simulink model "lqr_control"  (Simulink 8.0)
settings: Solver=FixedStepDiscrete  StartTime=0.0  StopTime=10.0  FixedStep=SampleTime  RelTol=1e-3
undefined symbols (not defined in the file or in its folder): DiscIntNeverNeededParam, K_pitch, K_roll, SampleTime
libraries: simulink x1
settings Model: Creator=austinmurch  LastModifiedBy=brtaylor
settings DataIOCC: SignalLoggingSaveFormat=ModelDataLogs
settings OptimizationCC: InlineParams=on  SimCompilerOptimization=On
settings DebuggingCC: FcnCallInpInsideContextMsg=UseLocalSettings  StrictBusMsg=Warning
settings HardwareCC: ProdLargestAtomicInteger=Long  ProdLargestAtomicFloat=Double  ProdIntDivRoundTo=Zero  ProdEndianess=BigEndian  ProdHWDeviceType=Freescale->32-bit PowerPC
settings ModelReferenceCC: ModelReferenceNumInstancesAllowed=Single
settings RTWCC: GenCodeOnly=on  GenerateMakefile=off  GenerateReport=on  CustomSourceCode="#include \"../../../Software/FlightCode/control/rtw_grt_control.c\""  LaunchReport=on
settings GRTTargetCC: CombineOutputUpdateFcns=off  GRTInterface=on

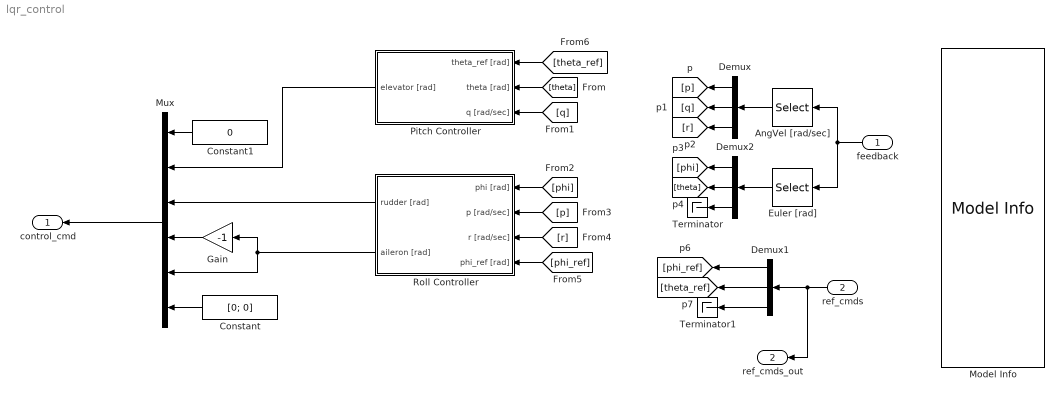
== system lqr_control ==
  feedback : Inport
  ref_cmds : Inport  Port=2
  AngVel [rad/sec] : Selector  InputPortWidth=19  IndexOptions=Index vector (dialog)  Indices=[4:6]  OutputSizes=1
  Constant : Constant  Value=[0; 0]
  Constant1 : Constant  Value=0
  Demux : Demux  Outputs=3
  Demux1 : Demux  Outputs=[1 1 10]
  Demux2 : Demux  Outputs=3
  Euler [rad] : Selector  InputPortWidth=19  IndexOptions=Index vector (dialog)  Indices=[1:3]  OutputSizes=1
  Gain : Gain  Gain=-1
  Model Info : simulink/Model-Wide Utilities/Model Info  InitialBlockCM=None  BlockCM=None  Frame=on  DisplayStringWithTags=|  HorizontalTextAlignment=Center  LeftAlignmentValue=0.5  SourceBlockDiagram=lqr_control  TagMaxNumber=20
      | Ref Cmd Port Info
      | 
      | 1. phi_cmd
      | 2. theta_cmd
      | 3. psi_cmd
      | 4. p_cmd
      | 5. q_cmd
      | 6. r_cmd
      | 7. V_s_cmd
      | 8. h_cmd
      | 9. gndtrk_cmd
      | 10. aoa_cmd
      | 11. aos_cmd
      | 12. gamma_cmd
      | 13. signal_0
      | 14. signal_1
      | 15. signal_2
      | 16. signal_3
      | 17. signal_4
      | 18. signal_5
      | 19. signal_6
      | 20. signal_7
      | 21. signal_8
      | 22. signal_9
  Mux : Mux  Inputs=6
  Pitch Controller : Subsystem
  Roll Controller : Subsystem
  Terminator : Terminator
  Terminator1 : Terminator
  control_cmd : Outport
  ref_cmds_out : Outport  Port=2
  wires:
  ref_cmds/1 -> ref_cmds_out/1, Demux1/1
  feedback/1 -> AngVel [rad/sec]/1, Euler [rad]/1
  AngVel [rad/sec]/1 -> Demux/1
  Euler [rad]/1 -> Demux2/1
  Demux/1 -> [p]
  Demux/2 -> [q]
  Demux/3 -> [r]
  Demux2/1 -> [phi]
  Demux2/2 -> [theta]
  Demux2/3 -> Terminator/1
  [theta] -> Pitch Controller/2(theta [rad])
  [q] -> Pitch Controller/3(q [rad/sec])
  [phi_ref] -> Roll Controller/4(phi_ref [rad])
  [r] -> Roll Controller/3(r [rad/sec])
  [p] -> Roll Controller/2(p [rad/sec])
  [phi] -> Roll Controller/1(phi [rad])
  [theta_ref] -> Pitch Controller/1(theta_ref [rad])
  Mux/1 -> control_cmd/1
  Pitch Controller/1(elevator [rad]) -> Mux/2
  Roll Controller/1(rudder [rad]) -> Mux/3
  Constant/1 -> Mux/6
  Constant1/1 -> Mux/1
  Roll Controller/2(aileron [rad]) -> Mux/5, Gain/1
  Gain/1 -> Mux/4
  Demux1/1 -> [phi_ref]
  Demux1/2 -> [theta_ref]
  Demux1/3 -> Terminator1/1

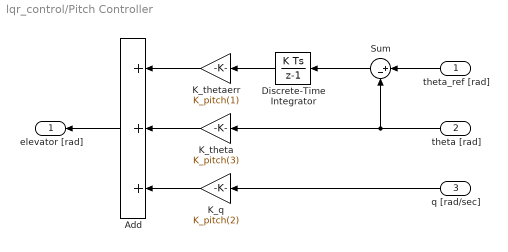
== system lqr_control/Pitch Controller ==
  theta_ref [rad] : Inport
  theta [rad] : Inport  Port=2
  q [rad/sec] : Inport  Port=3
  Add : Sum  Inputs=+++
  Discrete-Time Integrator : DiscreteIntegrator  SampleTime=SampleTime  ICPrevOutput=DiscIntNeverNeededParam  ICPrevScaledInput=DiscIntNeverNeededParam
  K_q : Gain  Gain=K_pitch(2)
  K_theta : Gain  Gain=K_pitch(3)
  K_thetaerr : Gain  Gain=K_pitch(1)
  Sum : Sum  Inputs=|+-
  elevator [rad] : Outport
  wires:
  Sum/1 -> Discrete-Time Integrator/1
  theta_ref [rad]/1 -> Sum/1
  theta [rad]/1 -> Sum/2, K_theta/1
  Discrete-Time Integrator/1 -> K_thetaerr/1
  q [rad/sec]/1 -> K_q/1
  K_thetaerr/1 -> Add/1
  K_theta/1 -> Add/2
  K_q/1 -> Add/3
  Add/1 -> elevator [rad]/1

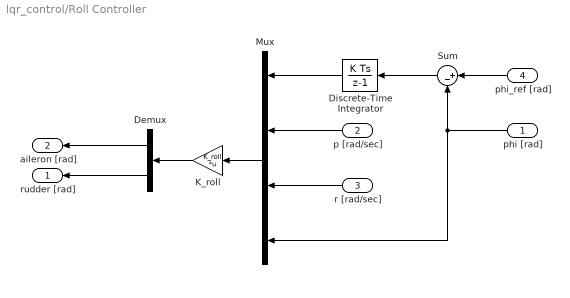
== system lqr_control/Roll Controller ==
  phi [rad] : Inport
  p [rad/sec] : Inport  Port=2
  r [rad/sec] : Inport  Port=3
  phi_ref [rad] : Inport  Port=4
  Demux : Demux  Outputs=2
  Discrete-Time Integrator : DiscreteIntegrator  SampleTime=SampleTime  ICPrevOutput=DiscIntNeverNeededParam  ICPrevScaledInput=DiscIntNeverNeededParam
  K_roll : Gain  Gain=K_roll  Multiplication=Matrix(K*u) (u vector)
  Mux : Mux
  Sum : Sum  Inputs=|+-
  rudder [rad] : Outport
  aileron [rad] : Outport  Port=2
  wires:
  p [rad/sec]/1 -> Mux/2
  Discrete-Time Integrator/1 -> Mux/1
  phi [rad]/1 -> Sum/2, Mux/4
  phi_ref [rad]/1 -> Sum/1
  Sum/1 -> Discrete-Time Integrator/1
  r [rad/sec]/1 -> Mux/3
  Mux/1 -> K_roll/1
  K_roll/1 -> Demux/1
  Demux/1 -> aileron [rad]/1
  Demux/2 -> rudder [rad]/1
